simulink model "simusink"  (R2018b)
settings: Solver=VariableStepAuto  StartTime=0.0  StopTime=5  FixedStep=0.1  RelTol=1e-3  EnableMultiTasking=on
values from neighbouring files (symbols this model uses):
  h0 = 0    [conversione_geodetic_ned.m]    (also in init_sensors.m)
  lat0 = 42.317744    [conversione_geodetic_ned.m]    (also in init_sensors.m)
  lon0 = 10.915136    [conversione_geodetic_ned.m]    (also in init_sensors.m)
  p_dvl = [0.2; 0 ; c]    [init_sensors.m]
  p_sonar_down = [0;0;c]    [init_sensors.m]
  p_sonar_front = [a;0;0]    [init_sensors.m]
  p_transponder = [50;60;36.4755]    [init_sensors.m]
  p_usbl = [-0.2; 0 ; c]    [init_sensors.m]
  tilt_down = deg2rad(0)    [init_sensors.m]
  tilt_front = deg2rad(45)    [init_sensors.m]
  Ts_ahrs = 0.05    [init_sensors.m]
  Ts_dvl = 1/7    (= 0.142857142857)    [init_sensors.m]
  Ts_giroscopio = 0.05    [init_sensors.m]
  Ts_gps = 1    [init_sensors.m]
  Ts_profondimetro = 0.05    [init_sensors.m]
  Ts_sonar_down = 0.5    [init_sensors.m]
  Ts_sonar_front = 0.5    [init_sensors.m]
  Ts_usbl = 2    [init_sensors.m]
  var_ahrs = [(deg2rad(0.1))^2; (deg2rad(0.1))^2; (deg2rad(1))^2]    [init_sensors.m]
  var_dvl = [(0.005^2); (0.005^2); (0.005^2)]    [init_sensors.m]
  var_giroscopio = [(deg2rad(0.16))^2;(deg2rad(0.16))^2;(deg2rad(0.16))^2]    [init_sensors.m]
  var_gps = [1;1;1]    [init_sensors.m]
  var_profondimetro = (0.05)^2    (= 0.0025)    [init_sensors.m]
  var_sonar_down = (0.15)^2    (= 0.0225)    [init_sensors.m]
  var_sonar_front = (0.15)^2    (= 0.0225)    [init_sensors.m]
  var_usbl = [(deg2rad(3)^2); (deg2rad(3))^2; (0.1)^2]    [init_sensors.m]
libraries: vrlib x1
settings Model: Creator=france  LastModifiedBy=chiara-s

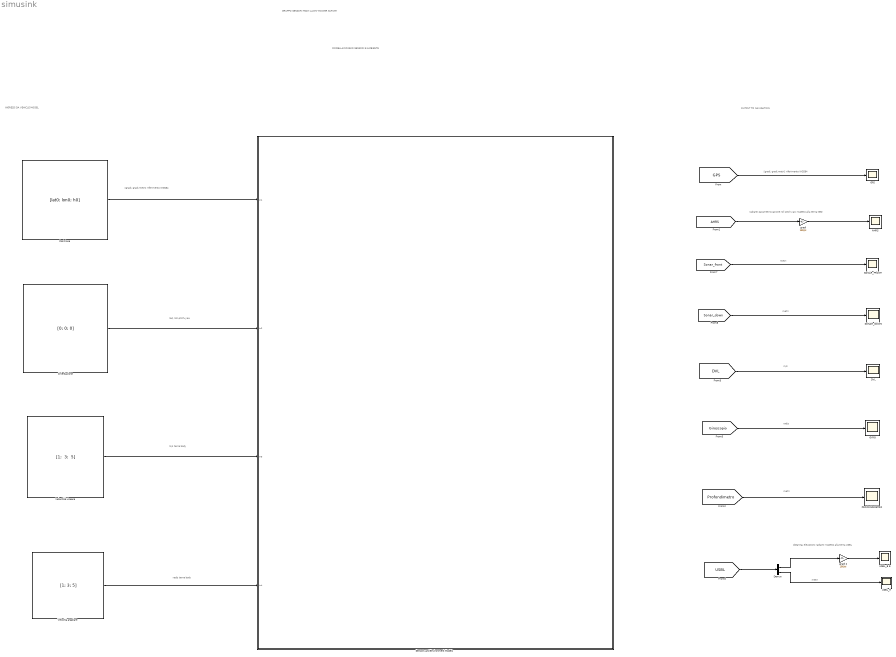
== system simusink ==
  note: rad, roll-pitch-yaw
  note: OUTPUT TO NAVIGATION
  note: metri
  note: [bearing, elevation] radianti rispetto alla terna USBL
  note: metri
  note: rad/s
  note: m/s
  note: metri
  note: m/s terna body
  note: rad/s terna body
  note: INGRESSI DA VEHICLE MODEL
  note: MODELLAZIONE DI SENSORI E AMBIENTE
  note: GRUPPO SENSORI TEAM LAWN-MOWER SURVEY
  note: [gradi, gradi,metri] riferimento WGS84
  note: radianti parametrizzazione roll pitch yaw rispetto alla terna NED
  note: metri
  note: [gradi, gradi,metri] riferimento WGS84
  " Velocità angolare" : Constant  Value=[1; 3; 5]  VectorParams1D=off  SampleTime=0.1
  AHRS : Scope
  DVL : Scope
  Demux : Demux  Outputs=2
  GPS : Scope
  GYRO : Scope
  Orientazione : Constant  Value=[0; 0; 0]  VectorParams1D=off  SampleTime=0.1
  PROFONDIMETRO : Scope
  Posizione : Constant  Value=[lat0; lon0; h0]  VectorParams1D=off
  SONAR_DOWN : Scope
  SONAR_FRONT : Scope
  "Sensors and Environment Models " : Subsystem
  USBL_B E : Scope
  "USBL_R " : Scope
  Velocitòà Lineare : Constant  Value="[1;  3;  5]"  VectorParams1D=off  SampleTime=0.1
  "gradi " : Gain  Gain=180/pi
  gradi 2 : Gain  Gain=180/pi
  wires:
  Demux/1 -> gradi 2/1
  Demux/2 -> "USBL_R "/1
  [Profondimetro] -> PROFONDIMETRO/1
  [AHRS] -> "gradi "/1
  [Sonar_front] -> SONAR_FRONT/1
  [Sonar_down] -> SONAR_DOWN/1
  [DVL] -> DVL/1
  [GPS] -> GPS/1
  [USBL] -> Demux/1
  "gradi "/1 -> AHRS/1
  [Giroscopio] -> GYRO/1
  gradi 2/1 -> USBL_B E/1
  Posizione/1 -> "Sensors and Environment Models "/1(In1)
  Orientazione/1 -> "Sensors and Environment Models "/2(In2)
  Velocitòà Lineare/1 -> "Sensors and Environment Models "/3(In3)
  " Velocità angolare"/1 -> "Sensors and Environment Models "/4(In4)

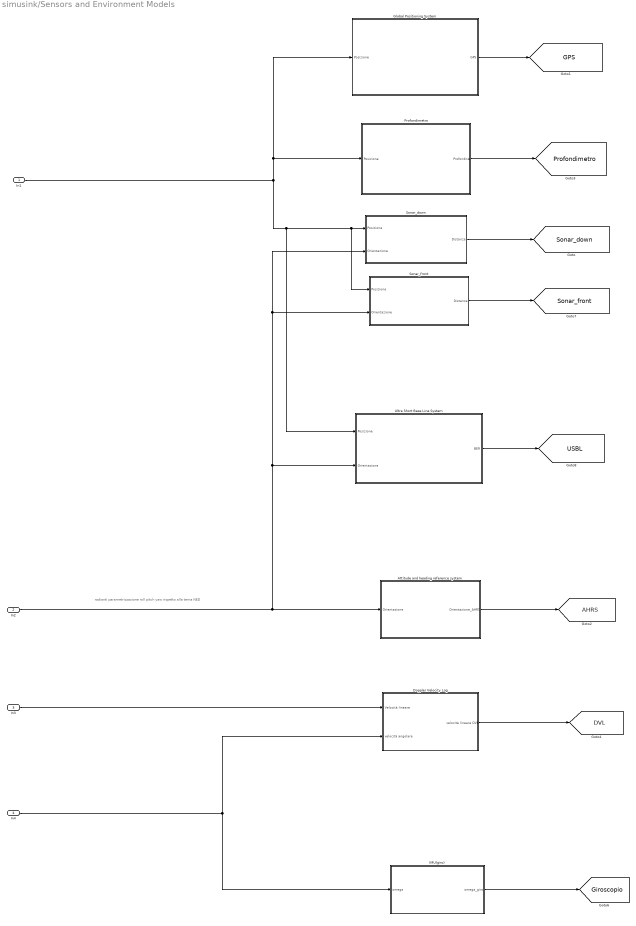
== system simusink/Sensors and Environment Models  ==
  note: radianti parametrizzazione roll pitch yaw rispetto alla terna NED
  In1 : Inport
  In2 : Inport  Port=2
  In3 : Inport  Port=3
  In4 : Inport  Port=4
  Attitude and heading reference system : Subsystem
  Doppler Velocity Log : Subsystem
  Global Positioning System : Subsystem
  IMU(giro) : Subsystem
  Profondimetro : Subsystem
  Sonar_down : Subsystem
  Sonar_front : Subsystem
  Ultra Short Base Line System : Subsystem
  tag scope: AHRS=global, DVL=global, GPS=global, Giroscopio=global, Profondimetro=global, Sonar_down=global, Sonar_front=global, USBL=global
  wires:
  Profondimetro/1(Profondità) -> [Profondimetro]
  IMU(giro)/1(omega_giro) -> [Giroscopio]
  Global Positioning System/1(GPS) -> [GPS]
  In3/1 -> Doppler Velocity Log/1(Velocità lineare)
  Sonar_front/1(Distanza) -> [Sonar_front]
  In1/1 -> Global Positioning System/1(Posizione), Profondimetro/1(Posizione), Ultra Short Base Line System/1(Posizione), Sonar_front/1(Posizione), Sonar_down/1(Posizione)
  In2/1 -> Sonar_down/2(Orientazione), Sonar_front/2(Orientazione), Ultra Short Base Line System/2(Orientazione), Attitude and heading reference system/1(Orientazione)
  Ultra Short Base Line System/1(BER) -> [USBL]
  In4/1 -> Doppler Velocity Log/2(velocità angolare), IMU(giro)/1(omega)
  Attitude and heading reference system/1(Orientazione_AHRS) -> [AHRS]
  Doppler Velocity Log/1(velocità lineare DVL) -> [DVL]
  Sonar_down/1(Distanza) -> [Sonar_down]

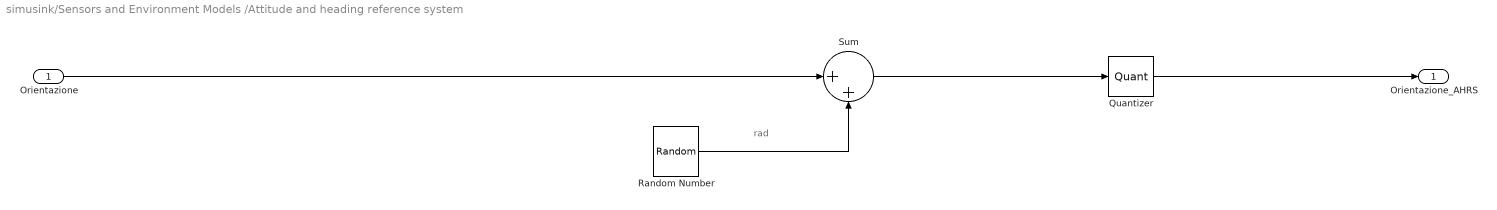
== system simusink/Sensors and Environment Models /Attitude and heading reference system ==
  note: rad
  Orientazione : Inport  SampleTime=Ts_ahrs
  Quantizer : Quantizer  QuantizationInterval=res_ahrs
  Random Number : RandomNumber  Variance=var_ahrs  Seed=[26; 78; 90]  SampleTime=Ts_ahrs  VectorParams1D=off
  Sum : Sum  Inputs=|++
  Orientazione_AHRS : Outport
  wires:
  Random Number/1 -> Sum/2
  Sum/1 -> Quantizer/1
  Orientazione/1 -> Sum/1
  Quantizer/1 -> Orientazione_AHRS/1

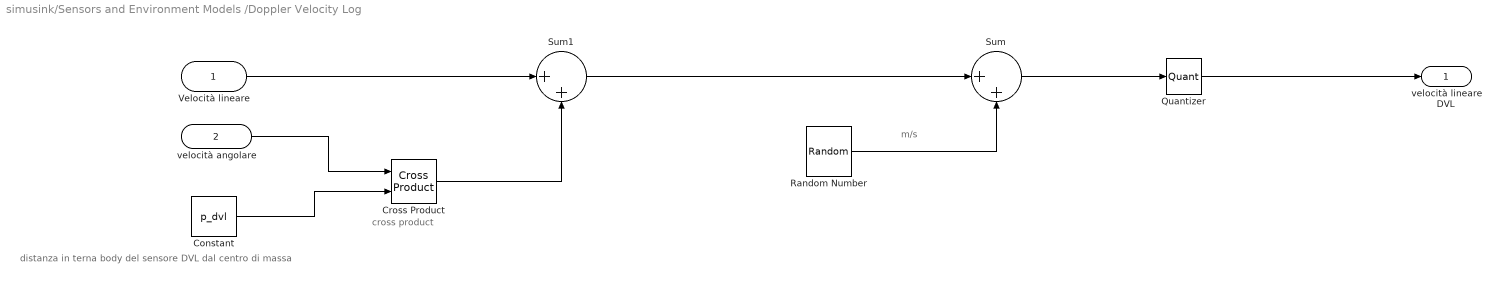
== system simusink/Sensors and Environment Models /Doppler Velocity Log ==
  note: distanza in terna body del sensore DVL dal centro di massa
  note: cross product
  note: m/s
  Velocità lineare : Inport  SampleTime=Ts_dvl
  velocità angolare : Inport  Port=2  SampleTime=Ts_dvl
  Constant : Constant  Value=p_dvl  VectorParams1D=off
  Cross Product : vrlib/Utilities/Cross Product
      settings: SourceProductBaseCode=VR
  Quantizer : Quantizer  QuantizationInterval=res_dvl
  Random Number : RandomNumber  Variance=var_dvl  Seed=[21, 68, 10]  SampleTime=Ts_dvl
  Sum : Sum  Inputs=|++
  Sum1 : Sum  Inputs=|++
  velocità lineare DVL : Outport
  wires:
  Sum/1 -> Quantizer/1
  Random Number/1 -> Sum/2
  velocità angolare/1 -> Cross Product/1
  Constant/1 -> Cross Product/2
  Velocità lineare/1 -> Sum1/1
  Cross Product/1 -> Sum1/2
  Sum1/1 -> Sum/1
  Quantizer/1 -> velocità lineare DVL/1

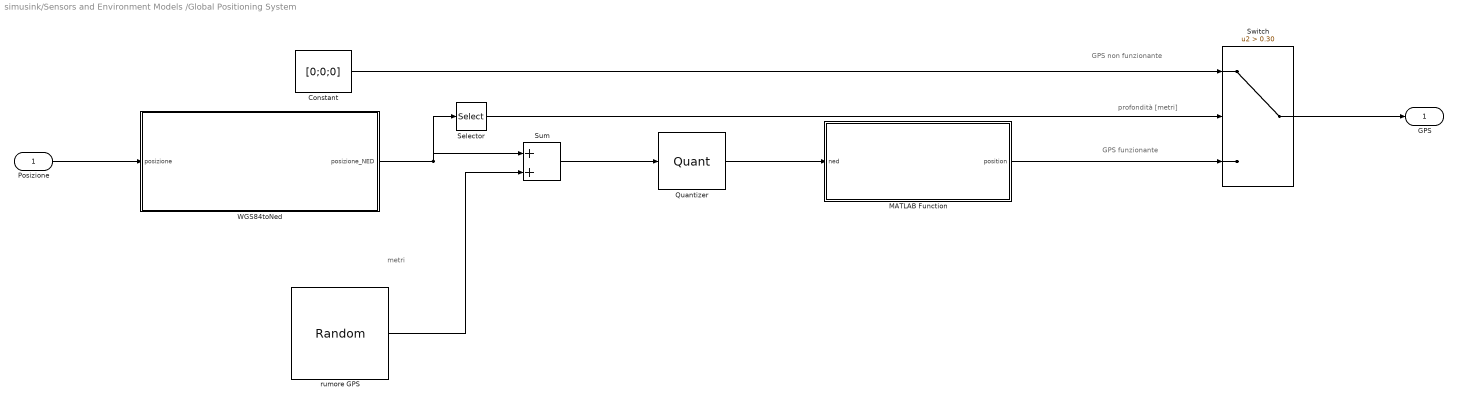
== system simusink/Sensors and Environment Models /Global Positioning System ==
  note: profondità [metri]
  note: GPS funzionante
  note: metri
  note: GPS non funzionante
  Posizione : Inport  SampleTime=Ts_gps
  Constant : Constant  Value=[0;0;0]  VectorParams1D=off
  MATLAB Function : MATLAB Function  TreatAsAtomicUnit=on
  Quantizer : Quantizer  QuantizationInterval=res_gps
  Selector : Selector  InputPortWidth=3  IndexOptions=Index vector (dialog)  Indices=[3]  OutputSizes=1
  Sum : Sum  Inputs=|++
  Switch : Switch  Criteria=u2 > Threshold  Threshold=0.30
  "WGS84toNed " : MATLAB Function  TreatAsAtomicUnit=on
  rumore GPS : RandomNumber  Variance=var_gps  Seed=[18;40;93]  SampleTime=Ts_gps  VectorParams1D=off
  GPS : Outport
  wires:
  Selector/1 -> Switch/2
  rumore GPS/1 -> Sum/2
  Posizione/1 -> "WGS84toNed "/1(posizione)
  "WGS84toNed "/1(posizione_NED) -> Selector/1, Sum/1
  Constant/1 -> Switch/1
  Sum/1 -> Quantizer/1
  MATLAB Function/1(position) -> Switch/3
  Switch/1 -> GPS/1
  Quantizer/1 -> MATLAB Function/1(ned)

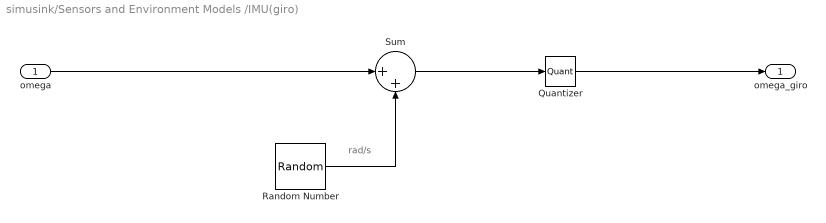
== system simusink/Sensors and Environment Models /IMU(giro) ==
  note: rad/s
  omega : Inport  SampleTime=Ts_giroscopio
  Quantizer : Quantizer  QuantizationInterval=res_giroscopio
  Random Number : RandomNumber  Variance=var_giroscopio  Seed=[1; 5; 3]  SampleTime=Ts_giroscopio  VectorParams1D=off
  Sum : Sum  Inputs=|++
  omega_giro : Outport
  wires:
  omega/1 -> Sum/1
  Random Number/1 -> Sum/2
  Sum/1 -> Quantizer/1
  Quantizer/1 -> omega_giro/1

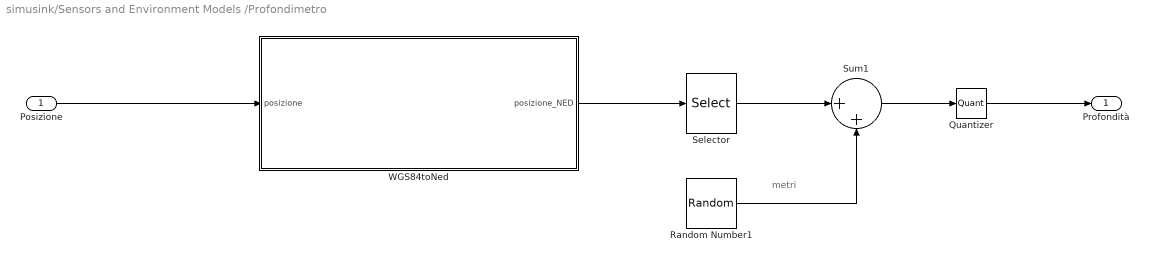
== system simusink/Sensors and Environment Models /Profondimetro ==
  note: metri
  Posizione : Inport  SampleTime=Ts_profondimetro
  Quantizer : Quantizer  QuantizationInterval=res_profondimetro
  Random Number1 : RandomNumber  Variance=var_profondimetro  Seed=85  SampleTime=Ts_profondimetro  VectorParams1D=off
  Selector : Selector  InputPortWidth=3  IndexOptions=Index vector (dialog)  Indices=[ 3]  OutputSizes=1
  Sum1 : Sum  Inputs=|++
  "WGS84toNed " : MATLAB Function  TreatAsAtomicUnit=on
  Profondità : Outport
  wires:
  Posizione/1 -> "WGS84toNed "/1(posizione)
  Selector/1 -> Sum1/1
  Random Number1/1 -> Sum1/2
  "WGS84toNed "/1(posizione_NED) -> Selector/1
  Sum1/1 -> Quantizer/1
  Quantizer/1 -> Profondità/1

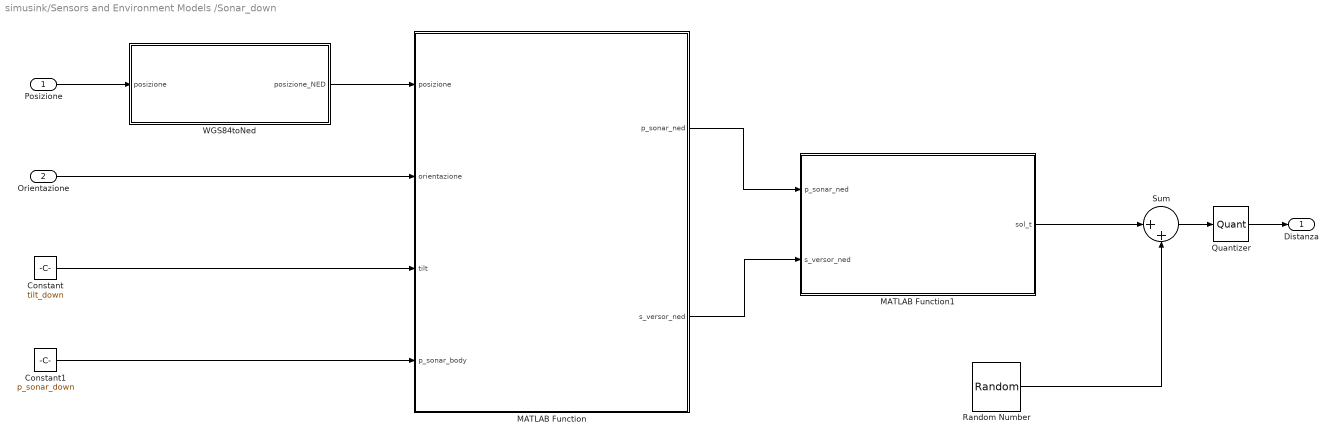
== system simusink/Sensors and Environment Models /Sonar_down ==
  Posizione : Inport  SampleTime=Ts_sonar_down
  Orientazione : Inport  Port=2  SampleTime=Ts_sonar_down
  Constant : Constant  Value=tilt_down  VectorParams1D=off  SampleTime=Ts_sonar_down
  Constant1 : Constant  Value=p_sonar_down  VectorParams1D=off  SampleTime=Ts_sonar_down
  MATLAB Function : MATLAB Function  TreatAsAtomicUnit=on
  MATLAB Function1 : MATLAB Function  TreatAsAtomicUnit=on
  Quantizer : Quantizer  QuantizationInterval=res_sonar_down
  Random Number : RandomNumber  Variance=var_sonar_down  SampleTime=Ts_sonar_down  VectorParams1D=off
  Sum : Sum  Inputs=|++
  "WGS84toNed " : MATLAB Function  TreatAsAtomicUnit=on
  Distanza : Outport
  wires:
  MATLAB Function/2(s_versor_ned) -> MATLAB Function1/2(s_versor_ned)
  "WGS84toNed "/1(posizione_NED) -> MATLAB Function/1(posizione)
  Constant1/1 -> MATLAB Function/4(p_sonar_body)
  MATLAB Function/1(p_sonar_ned) -> MATLAB Function1/1(p_sonar_ned)
  Orientazione/1 -> MATLAB Function/2(orientazione)
  Constant/1 -> MATLAB Function/3(tilt)
  Posizione/1 -> "WGS84toNed "/1(posizione)
  MATLAB Function1/1(sol_t) -> Sum/1
  Random Number/1 -> Sum/2
  Quantizer/1 -> Distanza/1
  Sum/1 -> Quantizer/1

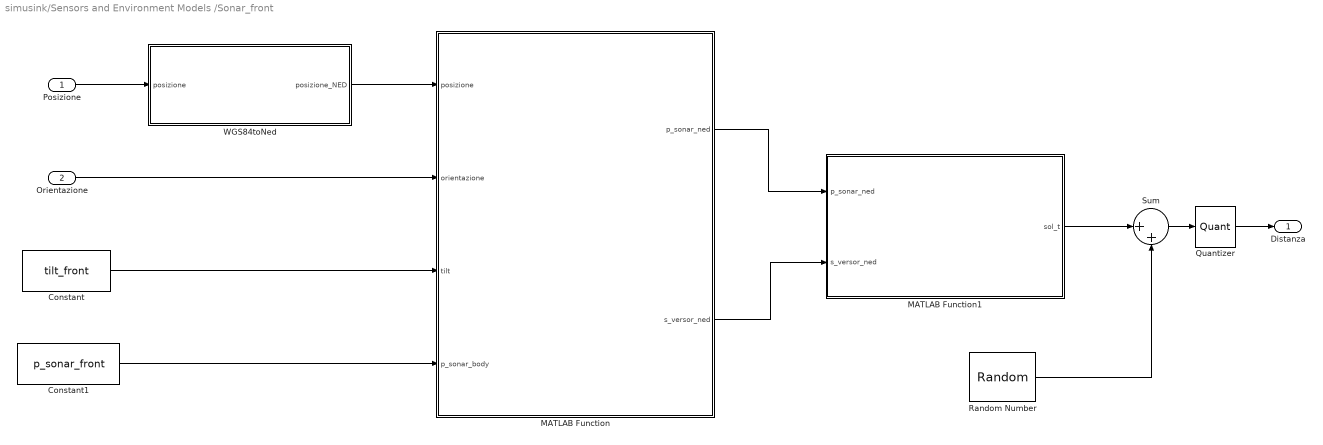
== system simusink/Sensors and Environment Models /Sonar_front ==
  Posizione : Inport  SampleTime=Ts_sonar_front
  Orientazione : Inport  Port=2  SampleTime=Ts_sonar_front
  Constant : Constant  Value=tilt_front  VectorParams1D=off  SampleTime=Ts_sonar_front
  Constant1 : Constant  Value=p_sonar_front  VectorParams1D=off  SampleTime=Ts_sonar_front
  MATLAB Function : MATLAB Function  TreatAsAtomicUnit=on
  MATLAB Function1 : MATLAB Function  TreatAsAtomicUnit=on
  Quantizer : Quantizer  QuantizationInterval=res_sonar_front
  Random Number : RandomNumber  Variance=var_sonar_front  SampleTime=Ts_sonar_front  VectorParams1D=off
  Sum : Sum  Inputs=|++
  "WGS84toNed " : MATLAB Function  TreatAsAtomicUnit=on
  Distanza : Outport
  wires:
  Posizione/1 -> "WGS84toNed "/1(posizione)
  Constant/1 -> MATLAB Function/3(tilt)
  Orientazione/1 -> MATLAB Function/2(orientazione)
  MATLAB Function/1(p_sonar_ned) -> MATLAB Function1/1(p_sonar_ned)
  Constant1/1 -> MATLAB Function/4(p_sonar_body)
  "WGS84toNed "/1(posizione_NED) -> MATLAB Function/1(posizione)
  MATLAB Function/2(s_versor_ned) -> MATLAB Function1/2(s_versor_ned)
  MATLAB Function1/1(sol_t) -> Sum/1
  Sum/1 -> Quantizer/1
  Random Number/1 -> Sum/2
  Quantizer/1 -> Distanza/1

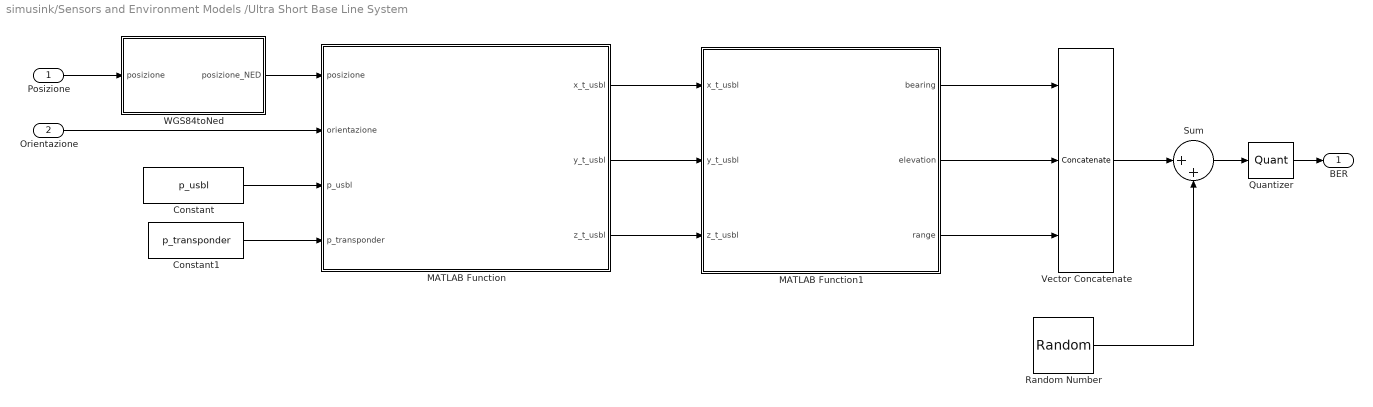
== system simusink/Sensors and Environment Models /Ultra Short Base Line System ==
  Posizione : Inport  SampleTime=Ts_usbl
  Orientazione : Inport  Port=2  SampleTime=Ts_usbl
  Constant : Constant  Value=p_usbl  VectorParams1D=off
  Constant1 : Constant  Value=p_transponder  VectorParams1D=off
  MATLAB Function : MATLAB Function  TreatAsAtomicUnit=on
  MATLAB Function1 : MATLAB Function  TreatAsAtomicUnit=on
  Quantizer : Quantizer  QuantizationInterval=res_usbl
  Random Number : RandomNumber  Variance=var_usbl  Seed=[2; 4; 1]  SampleTime=Ts_usbl  VectorParams1D=off
  Sum : Sum  Inputs=|++
  Vector Concatenate : Concatenate  NumInputs=3  Mode=Multidimensional array
  "WGS84toNed " : MATLAB Function  TreatAsAtomicUnit=on
  BER : Outport
  wires:
  MATLAB Function/1(x_t_usbl) -> MATLAB Function1/1(x_t_usbl)
  MATLAB Function1/2(elevation) -> Vector Concatenate/2
  Orientazione/1 -> MATLAB Function/2(orientazione)
  Constant/1 -> MATLAB Function/3(p_usbl)
  Constant1/1 -> MATLAB Function/4(p_transponder)
  Posizione/1 -> "WGS84toNed "/1(posizione)
  MATLAB Function1/1(bearing) -> Vector Concatenate/1
  MATLAB Function1/3(range) -> Vector Concatenate/3
  MATLAB Function/2(y_t_usbl) -> MATLAB Function1/2(y_t_usbl)
  "WGS84toNed "/1(posizione_NED) -> MATLAB Function/1(posizione)
  MATLAB Function/3(z_t_usbl) -> MATLAB Function1/3(z_t_usbl)
  Vector Concatenate/1 -> Sum/1
  Random Number/1 -> Sum/2
  Quantizer/1 -> BER/1
  Sum/1 -> Quantizer/1

== matlab function simusink/Sensors and Environment Models /Global Positioning System/MATLAB Function ==
  data: ned input; position output
function position = ned2wgs84(ned)

coder.extrinsic('evalin', 'ned2geodetic', 'wgs84Ellipsoid');
position = [0;0;0]
NED_origin = [0;0;0];
NED_origin = evalin('base', 'NED_origin');
[a b c] = ned2geodetic(ned(1), ned(2), ned(3), NED_origin(1), NED_origin(2),NED_origin(3), wgs84Ellipsoid);
position = [a; b; c]

end

== matlab function simusink/Sensors and Environment Models /Global Positioning System/WGS84toNed  ==
  data: posizione input; posizione_NED output
function posizione_NED = wgs84toNed(posizione)

coder.extrinsic('evalin', 'wgs84Ellipsoid', 'geodetic2ned');
NED_origin = [0;0;0];
posizione_NED  = [0;0;0];
NED_origin = evalin('base', 'NED_origin');
[a, b, c] = geodetic2ned(posizione(1), posizione(2), posizione(3), NED_origin(1), NED_origin(2), NED_origin(3), wgs84Ellipsoid);
posizione_NED = [a; b; c];

end

== matlab function simusink/Sensors and Environment Models /Profondimetro/WGS84toNed  ==
  data: posizione input; posizione_NED output
function posizione_NED = wgs84toNed(posizione)

coder.extrinsic('evalin', 'wgs84Ellipsoid', 'geodetic2ned');
NED_origin = [0;0;0];
posizione_NED  = [0;0;0];
NED_origin = evalin('base', 'NED_origin');
[a, b, c] = geodetic2ned(posizione(1), posizione(2), posizione(3), NED_origin(1), NED_origin(2), NED_origin(3), wgs84Ellipsoid);
posizione_NED = [a; b; c];

end

== matlab function simusink/Sensors and Environment Models /Sonar_down/MATLAB Function ==
  data: posizione input; p_sonar_ned output; orientazione input; s_versor_ned output; tilt input; p_sonar_body input
function [p_sonar_ned, s_versor_ned] = rot_body_ned(posizione,orientazione,tilt,p_sonar_body)
   
 roll = orientazione(1)
 pitch = orientazione(2)
 yaw = orientazione(3)
 xNorth = posizione(1)
 yEast = posizione(2)
 zDown = posizione(3)
 Rx = [1 0 0; 0 cos(roll) -sin(roll); 0 sin(roll) cos(roll)];
 Ry = [cos(pitch) 0 sin(pitch); 0 1 0; -sin(pitch) 0 cos(pitch)];
 Rz = [cos(yaw) -sin(yaw) 0; sin(yaw) cos(yaw) 0; 0 0 1];
 J1 = Rz*Ry*Rx; %matrice di rotazione da body a ned frame 

 s_versor_body = [sin(tilt); 0 ; cos(tilt)];	% direzione sonar in terna body
 s_versor_ned = J1*s_versor_body;
 
 cs2sensor_ned = J1*p_sonar_body; % distanza cds-sensore in Ned
 %Posizione sensore in Ned frame:
 p_sonar_ned = [xNorth; yEast; zDown] + cs2sensor_ned;
end

== matlab function simusink/Sensors and Environment Models /Sonar_down/MATLAB Function1 ==
  data: p_sonar_ned input; sol_t output; s_versor_ned input
function sol_t = sonar_down(p_sonar_ned, s_versor_ned)

coder.extrinsic('seabed_function');
sol_t = 0;
sol_t = seabed_function(p_sonar_ned, s_versor_ned)

end

== matlab function simusink/Sensors and Environment Models /Sonar_down/WGS84toNed  ==
  data: posizione input; posizione_NED output
function posizione_NED = wgs84toNed(posizione)

coder.extrinsic('evalin', 'wgs84Ellipsoid', 'geodetic2ned');
NED_origin = [0;0;0];
posizione_NED  = [0;0;0];
NED_origin = evalin('base', 'NED_origin');
[a, b, c] = geodetic2ned(posizione(1), posizione(2), posizione(3), NED_origin(1), NED_origin(2), NED_origin(3), wgs84Ellipsoid);
posizione_NED = [a; b; c];

end

== matlab function simusink/Sensors and Environment Models /Sonar_front/MATLAB Function ==
  data: posizione input; p_sonar_ned output; orientazione input; s_versor_ned output; tilt input; p_sonar_body input
function [p_sonar_ned, s_versor_ned] = rot_body_ned(posizione,orientazione,tilt,p_sonar_body)
   
 roll = orientazione(1)
 pitch = orientazione(2)
 yaw = orientazione(3)
 xNorth = posizione(1)
 yEast = posizione(2)
 zDown = posizione(3)
 Rx = [1 0 0; 0 cos(roll) -sin(roll); 0 sin(roll) cos(roll)];
 Ry = [cos(pitch) 0 sin(pitch); 0 1 0; -sin(pitch) 0 cos(pitch)];
 Rz = [cos(yaw) -sin(yaw) 0; sin(yaw) cos(yaw) 0; 0 0 1];
 J1 = Rz*Ry*Rx; %matrice di rotazione da body a ned frame 

 s_versor_body = [sin(tilt); 0 ; cos(tilt)];	% direzione sonar in terna body
 s_versor_ned = J1*s_versor_body;
 
 cs2sensor_ned = J1*p_sonar_body; % distanza cds-sensore in Ned
 %Posizione sensore in Ned frame:
 p_sonar_ned = [xNorth; yEast; zDown] + cs2sensor_ned;
end

== matlab function simusink/Sensors and Environment Models /Sonar_front/MATLAB Function1 ==
  data: p_sonar_ned input; sol_t output; s_versor_ned input
function sol_t = sonar_down(p_sonar_ned, s_versor_ned)

coder.extrinsic('seabed_function');
sol_t = 0;
sol_t = seabed_function(p_sonar_ned, s_versor_ned)

end

== matlab function simusink/Sensors and Environment Models /Sonar_front/WGS84toNed  ==
  data: posizione input; posizione_NED output
function posizione_NED = wgs84toNed(posizione)

coder.extrinsic('evalin', 'wgs84Ellipsoid', 'geodetic2ned');
NED_origin = [0;0;0];
posizione_NED  = [0;0;0];
NED_origin = evalin('base', 'NED_origin');
[a, b, c] = geodetic2ned(posizione(1), posizione(2), posizione(3), NED_origin(1), NED_origin(2), NED_origin(3), wgs84Ellipsoid);
posizione_NED = [a; b; c];

end

== matlab function simusink/Sensors and Environment Models /Ultra Short Base Line System/MATLAB Function ==
  data: posizione input; x_t_usbl output; orientazione input; p_usbl input; p_transponder input; y_t_usbl output; z_t_usbl output
function [x_t_usbl,y_t_usbl,z_t_usbl]= rot_ned_body(posizione,orientazione, p_usbl, p_transponder)
 
 roll = orientazione(1)
 pitch = orientazione(2)
 yaw = orientazione(3)
 xNorth = posizione(1)
 yEast = posizione(2)
 zDown = posizione(3)

 b2transp_ned = p_transponder-[xNorth;yEast;zDown]; %vettore distanza trasponder - veicolo espresso in ned 
 Rx = [1 0 0; 0 cos(roll) -sin(roll); 0 sin(roll) cos(roll)];
 Ry = [cos(pitch) 0 sin(pitch); 0 1 0; -sin(pitch) 0 cos(pitch)];
 Rz = [cos(yaw) -sin(yaw) 0; sin(yaw) cos(yaw) 0; 0 0 1];
 J1 = Rx'*Ry'*Rz'; %matrice di rotazione da ned a body frame 
 transponder_body = J1*b2transp_ned; %posizione transponder in terna body 
 transponder_usbl = transponder_body - p_usbl;  %posizione trasponder in terna usbl 
 x_t_usbl = transponder_usbl(1);
 y_t_usbl = transponder_usbl(2);
 z_t_usbl = transponder_usbl(3);
end

== matlab function simusink/Sensors and Environment Models /Ultra Short Base Line System/MATLAB Function1 ==
  data: x_t_usbl input; bearing output; y_t_usbl input; z_t_usbl input; elevation output; range output
function [bearing,elevation,range] = usbl(x_t_usbl, y_t_usbl, z_t_usbl)
 %coordinate sferiche in uscita dal sensore
 range = sqrt((x_t_usbl)^2+(y_t_usbl)^2+(z_t_usbl^2)); 
 elevation = asin(z_t_usbl/range);
 bearing = atan2(y_t_usbl,x_t_usbl); 

 end

== matlab function simusink/Sensors and Environment Models /Ultra Short Base Line System/WGS84toNed  ==
  data: posizione input; posizione_NED output
function posizione_NED = wgs84toNed(posizione)

coder.extrinsic('evalin', 'wgs84Ellipsoid', 'geodetic2ned');
NED_origin = [0;0;0];
posizione_NED  = [0;0;0];
NED_origin = evalin('base', 'NED_origin');
[a, b, c] = geodetic2ned(posizione(1), posizione(2), posizione(3), NED_origin(1), NED_origin(2), NED_origin(3), wgs84Ellipsoid);
posizione_NED = [a; b; c];

end
